simulink model "Exp_13"  (R2021a)
settings: Solver=VariableStepAuto  StartTime=0.0  StopTime=0.1  RelTol=1e-3
libraries: spsIGBTDiodeLib x4, spsSeriesRLCBranchLib x4, spsVoltageMeasurementLib x4, spsDCVoltageSourceLib x1, spsGroundLib x1, spspowerguiLib x1
settings Model: Creator=DCL  LastModifiedBy=DCL

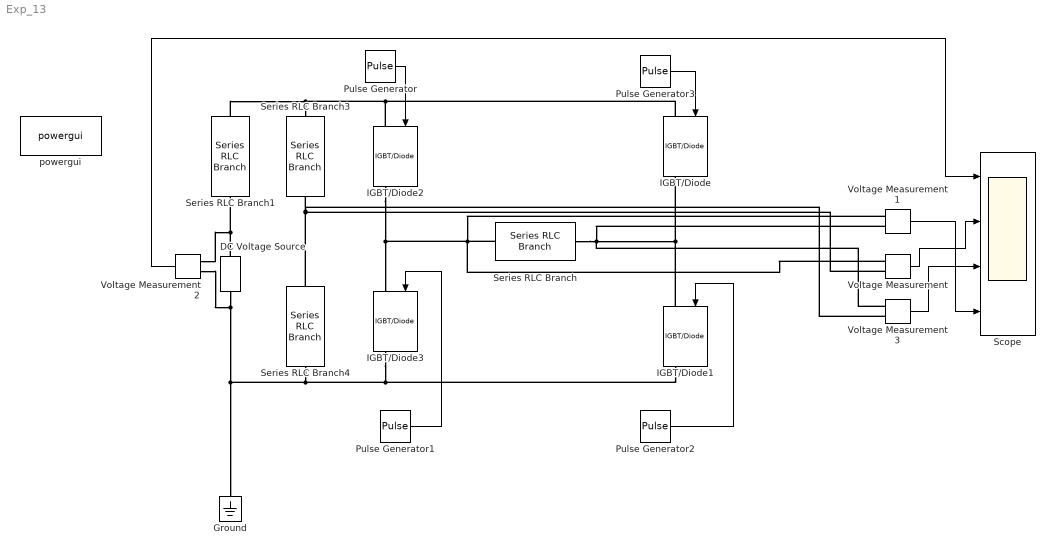
== system Exp_13 ==
  DC Voltage Source : spsDCVoltageSourceLib/DC Voltage Source  Amplitude=24  Measurements=None
  Ground : spsGroundLib/Ground  LConnTagsString=a
  IGBT/Diode{,1..3} (4 alike) : spsIGBTDiodeLib/IGBT//Diode  Ron=0.01  Rs=1e5  Cs=inf  Measurements=on
  Pulse Generator : DiscretePulseGenerator  PulseType=Time based  Period=0.02  PulseWidth=50  PhaseDelay=(0/360)*0.02
  Pulse Generator1 : DiscretePulseGenerator  PulseType=Time based  Period=0.02  PulseWidth=50  PhaseDelay=(180/360)* 0.02
  Pulse Generator2 : DiscretePulseGenerator  PulseType=Time based  Period=0.02  PulseWidth=50  PhaseDelay=(0/360)*0.02
  Pulse Generator3 : DiscretePulseGenerator  PulseType=Time based  Period=0.02  PulseWidth=50  PhaseDelay=(180/360)* 0.02
  Scope : Scope  NumInputPorts=4
  Series RLC Branch : spsSeriesRLCBranchLib/Series RLC Branch  LConnTagsString=__new0  RConnTagsString=__new0  BranchType=R  Resistance=10  Inductance=1e-3  SetiL0=off  InitialCurrent=0  Capacitance=1e-6  Setx0=off  InitialVoltage=0  Measurements=None
  Series RLC Branch1 : spsSeriesRLCBranchLib/Series RLC Branch  LConnTagsString=__new0  RConnTagsString=__new0  BranchType=R  Resistance=1  Inductance=1e-3  SetiL0=off  InitialCurrent=0  Capacitance=1e-6  Setx0=off  InitialVoltage=0  Measurements=None
  Series RLC Branch3 : spsSeriesRLCBranchLib/Series RLC Branch  LConnTagsString=__new0  RConnTagsString=__new0  BranchType=C  Resistance=1  Inductance=1e-3  SetiL0=off  InitialCurrent=0  Capacitance=0.1  Setx0=off  InitialVoltage=0  Measurements=None
  Series RLC Branch4 : spsSeriesRLCBranchLib/Series RLC Branch  LConnTagsString=__new0  RConnTagsString=__new0  BranchType=C  Resistance=1  Inductance=1e-3  SetiL0=off  InitialCurrent=0  Capacitance=0.1  Setx0=off  InitialVoltage=0  Measurements=None
  Voltage Measurement{,1..3} (4 alike) : spsVoltageMeasurementLib/Voltage Measurement  PhasorSimulation=off  OutputType=Complex  PSBequivalent=0
  powergui : spspowerguiLib/powergui  Priority=1  SimulationMode=Continuous  SampleTime=50e-6  frequency=60  Iterations=50  frequencyindice=0  Pbase=100e6  ErrMax=1e-4  UnitsV=kV  UnitsW=MW  buscounter=0  FunctionMessages=off  echomessages=off  EnableUseOfTLC=off  CurrentSourceSwitches=off  DisableSnubberDevices=off  DisableRonSwitches=off  DisableVfSwitches=off  DisplayEquations=off  AutomaticDiscreteSolvers=off  SolverType=Tustin/Backward Euler (TBE)  Interpol=off  ExternalGateDelay=off  methode=off  Ts=100  x0status=blocks  SPID=on  SwTol=0  HookPort=off  NonlinearTolerance=1e-4  nMaxIteration=100  ContinueOnMaxIteration=off  RestoreLinks=warning  ResistiveCurrentMeasurement=off  Frange=[0:2:500]  Ylog=off  Xlog=on  ShowGrid=off  save=off  variable=ZData  structure=0  ZoomFFT=off  StartTime=0.0  cycles=1  DisplayStyle=1  fundamental=60  FreqAxis=off  MaxFrequency=1000  frequencyindicesteady=1  RmsSteady=1  display=off
  wires:
  Pulse Generator/1 -> IGBT/Diode2/1
  Pulse Generator3/1 -> IGBT/Diode/1
  Pulse Generator1/1 -> IGBT/Diode3/1
  Pulse Generator2/1 -> IGBT/Diode1/1
  Voltage Measurement2/1 -> Scope/1
  Voltage Measurement1/1 -> Scope/4
  Voltage Measurement3/1 -> Scope/3
  Voltage Measurement/1 -> Scope/2
  connections:
  DC Voltage Source/RConn1 -- Series RLC Branch1/RConn1 -- Voltage Measurement2/LConn1
  DC Voltage Source/LConn1 -- IGBT/Diode1/RConn1 -- IGBT/Diode3/RConn1 -- Series RLC Branch4/RConn1 -- Ground/LConn1 -- Voltage Measurement2/LConn2
  Series RLC Branch1/LConn1 -- IGBT/Diode2/LConn1 -- IGBT/Diode/LConn1 -- Series RLC Branch3/LConn1
  Series RLC Branch4/LConn1 -- Voltage Measurement3/LConn2 -- Series RLC Branch3/RConn1 -- Voltage Measurement/LConn2
  IGBT/Diode2/RConn1 -- Voltage Measurement/LConn1 -- Voltage Measurement1/LConn1 -- Series RLC Branch/RConn1 -- IGBT/Diode3/LConn1
  IGBT/Diode1/LConn1 -- Voltage Measurement3/LConn1 -- Voltage Measurement1/LConn2 -- Series RLC Branch/LConn1 -- IGBT/Diode/RConn1
